simulink model "tank_pid_controller"  (R2013a)
settings: Solver=ode45  StartTime=0.0  StopTime=10  RelTol=1e-3
undefined symbols (not defined in the file): A, ka, ke, kv, n, R
libraries: simulink x1
settings Model: Creator=Ahmed  LastModifiedBy=Ahmed

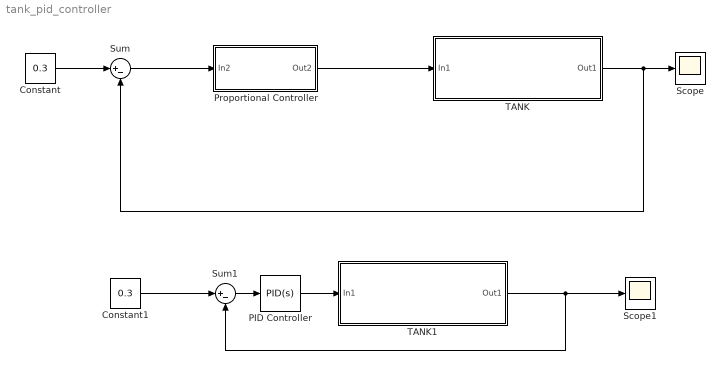
== system tank_pid_controller ==
  Constant : Constant  Value=0.3
  Constant1 : Constant  Value=0.3
  PID Controller : simulink/Continuous/PID Controller  Controller=PID  TimeDomain=Continuous-time  SampleTime=1  IntegratorMethod=Forward Euler  FilterMethod=Forward Euler  Form=Parallel  P=0  I=1667.47753388134  D=0  N=100  InitialConditionSource=internal  InitialConditionForIntegrator=0  InitialConditionForFilter=0  ExternalReset=none  LimitOutput=off  UpperSaturationLimit=inf  LowerSaturationLimit=-inf  LinearizeAsGain=on  AntiWindupMode=none  Kb=1  TrackingMode=off  Kt=1  PParamMin=[]  PParamMax=[]  IParamMin=[]  IParamMax=[]  DParamMin=[]  DParamMax=[]  NParamMin=[]  NParamMax=[]  KbParamMin=[]  KbParamMax=[]  KtParamMin=[]  KtParamMax=[]  POutMin=[]  POutMax=[]  IOutMin=[]  IOutMax=[]  DOutMin=[]  DOutMax=[]  NOutMin=[]  NOutMax=[]  KbOutMin=[]  KbOutMax=[]  KtOutMin=[]  KtOutMax=[]  IntegratorOutMin=[]  IntegratorOutMax=[]  FilterOutMin=[]  FilterOutMax=[]  SumOutMin=[]  SumOutMax=[]  SumI1OutMin=[]  SumI1OutMax=[]  SumI2OutMin=[]  SumI2OutMax=[]  SumI3OutMin=[]  SumI3OutMax=[]  SumDOutMin=[]  SumDOutMax=[]  SaturationOutMin=[]  SaturationOutMax=[]  IntegratorContinuousStateAttributes=''  IntegratorStateMustResolveToSignalObject=off  IntegratorRTWStateStorageClass=Auto  FilterContinuousStateAttributes=''  FilterStateMustResolveToSignalObject=off  FilterRTWStateStorageClass=Auto
  Proportional Controller : Subsystem
  Scope : Scope
  Scope1 : Scope
  Sum : Sum  Inputs=|+-
  Sum1 : Sum  Inputs=|+-
  TANK : Subsystem
  TANK1 : Subsystem
  wires:
  TANK/1(Out1) -> Sum/2, Scope/1
  Constant/1 -> Sum/1
  Sum/1 -> Proportional Controller/1(In2)
  Proportional Controller/1(Out2) -> TANK/1(In1)
  TANK1/1(Out1) -> Scope1/1, Sum1/2
  Sum1/1 -> PID Controller/1
  PID Controller/1 -> TANK1/1(In1)
  Constant1/1 -> Sum1/1

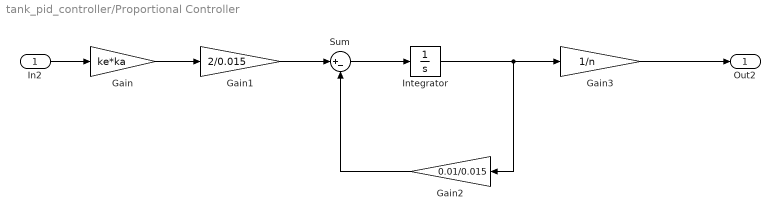
== system tank_pid_controller/Proportional Controller ==
  In2 : Inport
  Gain : Gain  Gain=ke*ka
  Gain1 : Gain  Gain=2/0.015
  Gain2 : Gain  Gain=0.01/0.015
  Gain3 : Gain  Gain=1/n
  Integrator : Integrator
  Sum : Sum  Inputs=|+-
  Out2 : Outport
  wires:
  In2/1 -> Gain/1
  Gain/1 -> Gain1/1
  Gain1/1 -> Sum/1
  Sum/1 -> Integrator/1
  Integrator/1 -> Gain3/1, Gain2/1
  Gain2/1 -> Sum/2
  Gain3/1 -> Out2/1

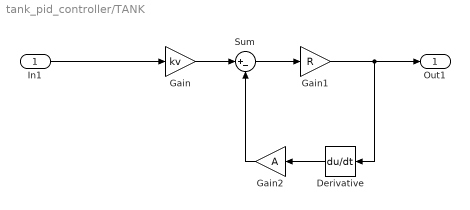
== system tank_pid_controller/TANK ==
  In1 : Inport
  Derivative : Derivative
  Gain : Gain  Gain=kv
  Gain1 : Gain  Gain=R
  Gain2 : Gain  Gain=A
  Sum : Sum  Inputs=|+-
  Out1 : Outport
  wires:
  Derivative/1 -> Gain2/1
  Gain/1 -> Sum/1
  Gain1/1 -> Out1/1, Derivative/1
  In1/1 -> Gain/1
  Sum/1 -> Gain1/1
  Gain2/1 -> Sum/2

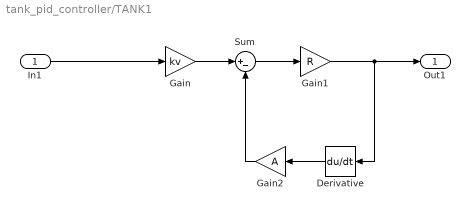
== system tank_pid_controller/TANK1 ==
  In1 : Inport
  Derivative : Derivative
  Gain : Gain  Gain=kv
  Gain1 : Gain  Gain=R
  Gain2 : Gain  Gain=A
  Sum : Sum  Inputs=|+-
  Out1 : Outport
  wires:
  Gain2/1 -> Sum/2
  Sum/1 -> Gain1/1
  In1/1 -> Gain/1
  Gain1/1 -> Derivative/1, Out1/1
  Gain/1 -> Sum/1
  Derivative/1 -> Gain2/1
